simulink model "simulink_model_advanced_closed_loop_with_param"  (R2020a)
settings: Solver=ode45  StartTime=0.0  StopTime=2  RelTol=1e-3
values from neighbouring files (symbols this model uses):
  N = 20    [minimal_example_closed_loop.m]    (also in minimal_example_ocp_with_param.m)
  nu = model.nu    [minimal_example_closed_loop.m]    (also in minimal_example_ocp_with_param.m)
  nx = model.nx    [minimal_example_closed_loop.m]    (also in minimal_example_ocp_with_param.m)
  ny = size(model.cost_expr_y, 1)    [minimal_example_closed_loop.m]    (also in minimal_example_ocp_with_param.m)
  ny_e = size(model.cost_expr_y_e, 1)    [minimal_example_closed_loop.m]    (also in minimal_example_ocp_with_param.m)
  U_max = 80    [minimal_example_closed_loop.m]    (also in minimal_example_ocp_with_param.m)
  x0 = x_sim(:,i)    [minimal_example_closed_loop.m]    (also in minimal_example_ocp_with_param.m = [0; pi; 0; 0])
settings Model: Creator=oj  LastModifiedBy=sandmann
settings DataIOCC: SaveFormat=StructureWithTime
settings OptimizationCC: LifeSpan=inf
settings DebuggingCC: SFExecutionAtInitializationDiag=none  ArithmeticOperatorsInVariantConditions=warning
settings HardwareCC: ProdBitPerSizeT=32  ProdBitPerPtrDiffT=32  ProdWordSize=32  ProdHWDeviceType=Specified
settings SFSimCC: CustomCodeUndefinedFunction=UseInterfaceOnly
settings CodeAppCC: StateflowObjectComments=on

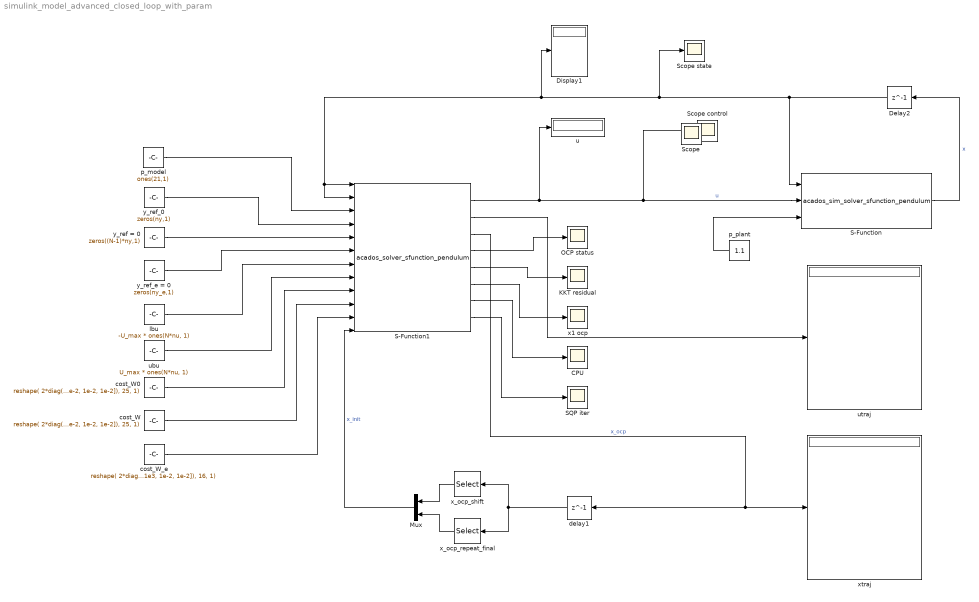
== system simulink_model_advanced_closed_loop_with_param ==
  CPU : Scope
      settings: Description=status
  Delay2 : Delay  DelayLength=1  InitialCondition=x0
  Display1 : Display
  KKT residual : Scope
      settings: Description=status
  Mux : Mux  Inputs=2
  OCP status : Scope
      settings: Description=status
  S-Function : S-Function  FunctionName=acados_sim_solver_sfunction_pendulum  SFunctionDeploymentMode=off  EnableBusSupport=off
  S-Function1 : S-Function  FunctionName=acados_solver_sfunction_pendulum  SFunctionDeploymentMode=off  EnableBusSupport=off
  SQP iter : Scope
      settings: Description=status
  Scope control : Scope
  Scope state : Scope
  cost_W : Constant  Value=reshape( 2*diag([1e3, 1e3, 1e-2, 1e-2, 1e-2]), 25, 1)
  cost_W0 : Constant  Value=reshape( 2*diag([1e3, 1e3, 1e-2, 1e-2, 1e-2]), 25, 1)
  cost_W_e : Constant  Value=reshape( 2*diag([1e3, 1e3, 1e-2, 1e-2]), 16, 1)
  delay1 : Delay  DelayLength=1  InitialCondition=zeros(nx*(N+1),1)
  lbu : Constant  Value=-U_max * ones(N*nu, 1)
  p_model : Constant  Value=ones(21,1)
  p_plant : Constant  Value=1.1
  u : Display
  ubu : Constant  Value=U_max * ones(N*nu, 1)
  utraj : Display
  x1 ocp : Scope
      settings: Description=status
  x_ocp_repeat_final : Selector  IndexMode=Zero-based  InputPortWidth=(N+1)*nx  IndexOptions=Starting index (dialog)  Indices=N*nx  OutputSizes=nx
  x_ocp_shift : Selector  IndexMode=Zero-based  InputPortWidth=(N+1)*nx  IndexOptions=Starting index (dialog)  Indices=nx  OutputSizes=N*nx
  xtraj : Display
  y_ref = 0 : Constant  Value=zeros((N-1)*ny,1)
  y_ref_0 : Constant  Value=zeros(ny,1)
  y_ref_e = 0 : Constant  Value=zeros(ny_e,1)
  Scope : Scope
  wires:
  S-Function/1 -> Delay2/1  "x"
  S-Function1/4 -> OCP status/1
  S-Function1/5 -> KKT residual/1
  S-Function1/6 -> x1 ocp/1
  S-Function1/7 -> CPU/1
  y_ref = 0/1 -> S-Function1/5
  y_ref_e = 0/1 -> S-Function1/6
  lbu/1 -> S-Function1/7
  ubu/1 -> S-Function1/8
  S-Function1/1 -> u/1, Scope control/1, S-Function/2  "u"
  Delay2/1 -> Scope state/1, Display1/1, S-Function1/2, S-Function1/1, S-Function/1
  S-Function1/8 -> SQP iter/1
  cost_W0/1 -> S-Function1/9
  cost_W/1 -> S-Function1/10
  cost_W_e/1 -> S-Function1/11
  y_ref_0/1 -> S-Function1/4
  S-Function1/2 -> utraj/1
  x_ocp_shift/1 -> Mux/1
  delay1/1 -> x_ocp_shift/1, x_ocp_repeat_final/1
  Mux/1 -> S-Function1/12  "x_init"
  x_ocp_repeat_final/1 -> Mux/2
  S-Function1/3 -> xtraj/1, delay1/1  "x_ocp"
  p_model/1 -> S-Function1/3
  p_plant/1 -> S-Function/3
